simulink model "variableselector_tut"  (Simulink 4.00)
settings: Solver=FixedStepDiscrete  StartTime=0.0  StopTime=10.0  RelTol=1e-3
PreLoadFcn:
  | dsp_examples_A = [1:10;1 1 0 0 1 1 0 0 1 1]';
PostLoadFcn:
  | set_param(gcs,'SimulationCommand','Update')
libraries: dspindex x1, dspsrcs3 x1
settings Model: RequirementInfo=9  Creator=ckamachi  LastModifiedBy=ckamachi  LimitDataPoints=off  ExtModeTrigMode=oneshot  ExtModeArmWhenConnect=off  BlockReductionOpt=off

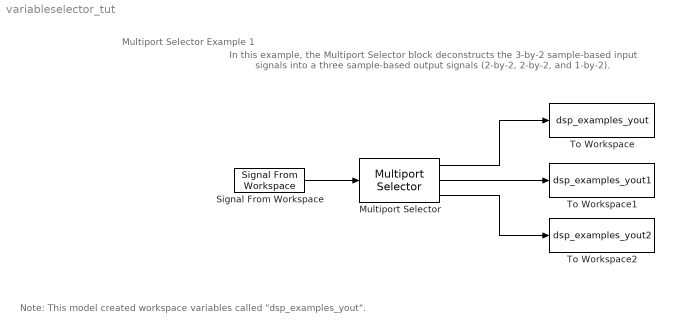
== system variableselector_tut ==
  note: Multiport Selector Example 1
  note: In this example, the Multiport Selector block deconstructs
      | the 3-by-2 sample-based input signals into a three
      | sample-based output signals (2-by-2, 2-by-2, and 1-by-2).
  note: Note: This model created workspace variables called "dsp_examples_yout".
  Multiport Selector : dspindex/Multiport Selector  rowsOrCols=Rows  idxCellArray={ [1 2], [1 3], 3 }  idxErrMode=Clip Index
  Signal From Workspace : dspsrcs3/Signal From Workspace  X=randn(3,2,10)  Ts=1  nsamps=1  OutputAfterFinalValue=Setting To Zero
  To Workspace : ToWorkspace  VariableName=dsp_examples_yout  SampleTime=-1  SaveFormat=Array
  To Workspace1 : ToWorkspace  VariableName=dsp_examples_yout1  SampleTime=-1  SaveFormat=Array
  To Workspace2 : ToWorkspace  VariableName=dsp_examples_yout2  SampleTime=-1  SaveFormat=Array
  wires:
  Signal From Workspace/1 -> Multiport Selector/1
  Multiport Selector/1 -> To Workspace/1
  Multiport Selector/2 -> To Workspace1/1
  Multiport Selector/3 -> To Workspace2/1
